simulink model "RadarSimulinkProjectRev003"  (R2024a)
settings: Solver=VariableStepAuto  StartTime=0.0  StopTime=0.012  RelTol=1e-3
values from neighbouring files (symbols this model uses):
  AngleTime = SweepTime/10    (= 10000)    [InitializationOfVariablesRev000.m]    (also in InitializationOfVariablesRev001.m; InitializationOfVariablesRev002.m = 2000; InitializationOfVariablesRev003.m = 20000; InitializationOfVariablesRev004.m = 2097152)
  ASR_LUT = Rsamp    [InitializationOfVariablesRev003.m]    (also in InitializationOfVariablesRev004.m = round((R*2*SystemFs)/c); InitializationOfVariablesRev005.m = round((R*2*SystemFs)/c))
  Btn_Debounce = 20000    [InitializationOfVariablesRev003.m]    (also in InitializationOfVariablesRev004.m; InitializationOfVariablesRev005.m)
  ChirpNc = 128    [InitializationOfVariablesRev004.m]    (also in InitializationOfVariablesRev005.m)
  ChirpSizeLength = length(FCW)    [InitializationOfVariablesRev004.m]    (also in InitializationOfVariablesRev005.m = 16384)
  FreqDeltaPeriod = 54    [InitializationOfVariablesRev003.m]    (also in InitializationOfVariablesRev004.m = 1)
  RXFFTLength = 4096    [InitializationOfVariablesRev003.m]    (also in InitializationOfVariablesRev004.m = 1024; InitializationOfVariablesRev005.m = 2048)
  SweepTime = 100000    [InitializationOfVariablesRev000.m]    (also in InitializationOfVariablesRev001.m; InitializationOfVariablesRev002.m = 20000; InitializationOfVariablesRev003.m = 200000; InitializationOfVariablesRev004.m = 23068672)
undefined symbols (not defined in the file or in its folder): SignalGenerationForAnalysis, Subsystem, xc7a200tfbg676
libraries: hdlBasic x247, hdlDSPIP x12, hdlUtilities x2, vmcUtilities x1
(part 1 of 2)
settings Model: Creator=Cube II  LastModifiedBy=Cube II

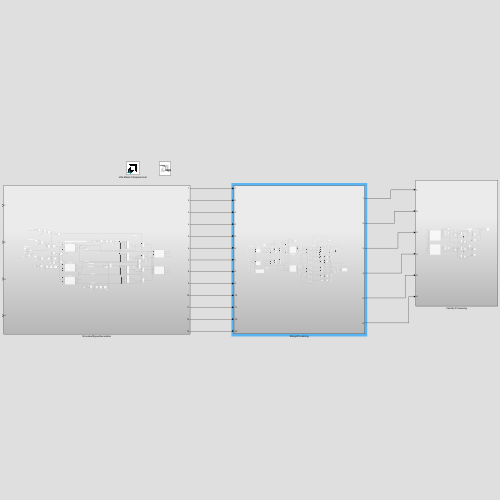
[thumbnail: Simulink's stored preview of the top-level diagram]
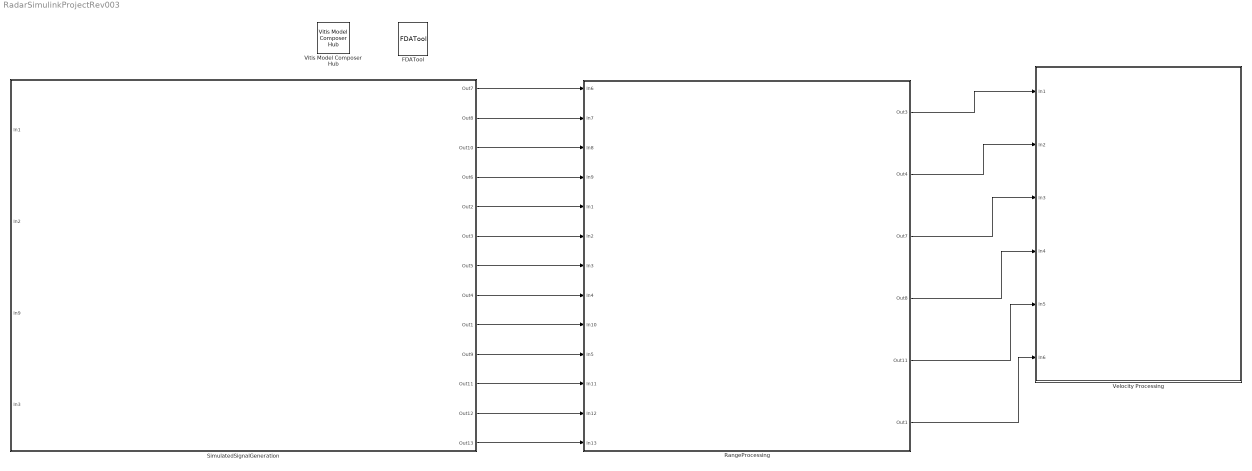
== system RadarSimulinkProjectRev003 ==
  FDATool : hdlUtilities/FDATool  block_type=fdatool
      settings: infoedit=FDATool
  RangeProcessing : Subsystem
  SimulatedSignalGeneration : Subsystem  SystemSampleTime=1/200e6
  Velocity Processing : Subsystem
  Vitis Model Composer Hub : vmcUtilities/Vitis Model Composer Hub  Tag=genX  CodeGeneration=off  SubsystemName=Subsystem  BlockHierPath=SignalGenerationForAnalysis/Subsystem  CompilationType=HDLCompilation  SubsystemType=HDLNode  ExportTypeV2=IP Catalog  StartColumn=1  NumberOfColumns=1  TargetDirectory=./netlist  exportDesign=off  analyzeDesign=on  validateDesignOnHw=off  ExportType=AI Engines  IpVendor=xilinx.com  IpLibrary=hls  IpVersion=1.0  IpHWLanguage=Verilog  AieCompilerOptions={}  AieSimulatorOptions={}  CreateTestbench=on  TestbenchStackSize=10  RunRtlSim=off  RunCSim=off  RunAieSim=off  AieSimTimeout=50000  RunAieSimProfiling=off  LaunchVitisAnalyzer=off  PlotOutput=off  RunX86Sim=off  X86SimTimeout=10  GenHwImage=off  GenLibadfXo=on  GenHwValidationCode=off  PlatformType=Not Specified  HwSystemType=Baremetal  HwValidationTarget=hw  ProjDevice=Artix-7 AC701 Evaluation Platform (xc7a200tfbg676-2)  ProjDevicePart=xc7a200tfbg676-2  AIEType=None  SamplePeriod=-1  ClockFrequency=200  DataPathParallelism=1  xilinxfamily=artix7  part=xc7a200t  speed=-2  package=fbg676  directory=./netlist\ip\Subsystem\src  testbench=off  incr_netlist=off  synthesis_tool=Vivado  clock_wrapper=Clock Enables  dbl_ovrd=According to Block Masks  dcm_input_clock_period=10  sysclk_period=5  simulink_period=1/200e6  eval_field=0  IPInfoJsonString="{\"DUTSubsystemName\":\"Subsystem\",\"HDLSubsystem\":{\"SubsystemName\":\"Subsystem\",\"IPName\":\"Subsystem\",\"IPLibrary\":\"VMC\",\"IPVendor\":\"User Company\",\"IPVersion\":\"1.0\",\"TargetDirectory\":\"./netlist\",\"SubsystemDir\":\"./netlist\\\\ip\\\\Subsystem\",\"FreqHz\":\"200000000\"},\"SubsystemTag\":\"HDLNode\"}"  LogFileName=S:\RadarProjectSimulink\netlist\model_composer.log  NThreads=4  IPConfigFile=C:\Users\Cube II\AppData\Local\Temp\vmctmp-5941030035629153029\SignalGenerationForAnalysis_ipconfig.json
  wires:
  SimulatedSignalGeneration/3(Out10) -> RangeProcessing/3(In8)
  SimulatedSignalGeneration/4(Out6) -> RangeProcessing/4(In9)
  SimulatedSignalGeneration/7(Out5) -> RangeProcessing/7(In3)
  SimulatedSignalGeneration/8(Out4) -> RangeProcessing/8(In4)
  SimulatedSignalGeneration/10(Out9) -> RangeProcessing/10(In5)
  SimulatedSignalGeneration/9(Out1) -> RangeProcessing/9(In10)
  SimulatedSignalGeneration/2(Out8) -> RangeProcessing/2(In7)
  SimulatedSignalGeneration/1(Out7) -> RangeProcessing/1(In6)
  SimulatedSignalGeneration/6(Out3) -> RangeProcessing/6(In2)
  SimulatedSignalGeneration/5(Out2) -> RangeProcessing/5(In1)
  SimulatedSignalGeneration/11(Out11) -> RangeProcessing/11(In11)
  SimulatedSignalGeneration/12(Out12) -> RangeProcessing/12(In12)
  RangeProcessing/1(Out3) -> Velocity Processing/1(In1)
  RangeProcessing/2(Out4) -> Velocity Processing/2(In2)
  RangeProcessing/3(Out7) -> Velocity Processing/3(In3)
  RangeProcessing/4(Out8) -> Velocity Processing/4(In4)
  RangeProcessing/5(Out11) -> Velocity Processing/5(In5)
  RangeProcessing/6(Out1) -> Velocity Processing/6(In6)
  SimulatedSignalGeneration/13(Out13) -> RangeProcessing/13(In13)

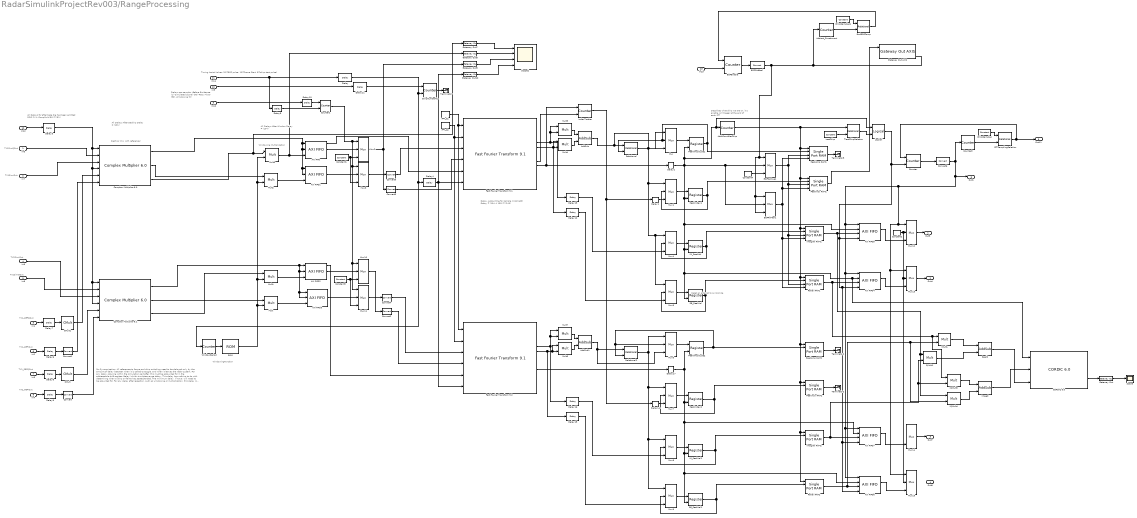
== system RadarSimulinkProjectRev003/RangeProcessing ==
  note: Describes what chirp we are on, it's enable will trigger at the end of each FFT
  note: All Delays for after base Sig has been emitted
      | DDS (1) + CompMult (50) = (51)
  note: Delays per sample:
      | -Before Emittance (1)
      | -Simulated Signal (50)
      | -Recv Mixer (50)
      | -Windowing (3)
  note: TX1SimIOut
  note: TX1SimQOut
  note: TX2SimIOut
  note: TX2SimQOut
  note: TX1_REFIOut
  note: TX1_REFQOut
  note: TX2_REFIOut
  note: TX1_REFQOut
  note: Dechirp (mix with reference)
  note: Timing Assist Values (11=EOF pulse, 10=Frame Start, 9=chirp start pulse)
  note: WindowingFunction
  note: Windowing Multiplication
  note: For Syncronization: All references to frame and chirp switching need to be delayed only by the amount of delay between when it is called to toggle, and when it leaves the radar system.
      |
      | For any delay occuring within the simulation part after, this must be accounted for in the addressable shift register (delay) which simulates range delay. This delay has nothing to do with determinng when a chirp or frame has started/ended. The minimum delay, if not 0, will need to be acounted for.
      |
      | For any delay after reception, such as windowing or multiplication, this delay is relevant to anything that has to do with the processes that depend on knowing when a frame or chirp has started/ended. Since it should only start sampling once a signal theoretically should have arrived from 0 meters (no sim delay)
  note: All Delays After Dechirp
      | Delay = (101)
  note: Delay, accounting for sample missmatch
      | Delay = (104 + 139) = (243)
  note: All Delays After Window
      | Delay = (104)
  note: Reset an attempt to syncronize
  In6 : Inport
  In7 : Inport  Port=2
  In8 : Inport  Port=3
  In9 : Inport  Port=4
  In1 : Inport  Port=5
  In2 : Inport  Port=6
  In3 : Inport  Port=7
  In4 : Inport  Port=8
  In10 : Inport  Port=9
  In5 : Inport  Port=10
  In11 : Inport  Port=11
  In12 : Inport  Port=12
  In13 : Inport  Port=13
  AXI FIFO{,1..3} (4 alike) : hdlBasic/AXI FIFO  input_depth_axis=256  actual_fifo_depth_label=258  enable_tdata=on  enable_tdest=off  enable_tstrb=off  enable_tready=on  enable_tid=off  enable_tuser=off  enable_tkeep=off  enable_tlast=off  has_aresetn=off  enable_data_counts_axis=off  fifo_implementation_type_axis=Common Clock Block RAM  trim_axipin_name=on  programmable_full_type_axis=Full  full_threshold_assert_value_axis=0  programmable_empty_type_axis=Empty  empty_threshold_assert_value_axis=1022  underflow_flag_axi=0  underflow_sense_axi=Active High  overflow_flag_axi=0  overflow_sense_axi=Active High  simulation_type=fast_sim  XmcBlockStatus=1  maskContainerNames=tabcontainer1  block_type=axi_fifo  block_config=sysgen:AXI_FIFO_config
  AXI FIFO{4..7} (4 alike) : hdlBasic/AXI FIFO  input_depth_axis=128  actual_fifo_depth_label=130  enable_tdata=on  enable_tdest=off  enable_tstrb=off  enable_tready=on  enable_tid=off  enable_tuser=off  enable_tkeep=off  enable_tlast=on  has_aresetn=off  enable_data_counts_axis=off  fifo_implementation_type_axis=Common Clock Block RAM  trim_axipin_name=on  programmable_full_type_axis=Full  full_threshold_assert_value_axis=0  programmable_empty_type_axis=Empty  empty_threshold_assert_value_axis=1022  underflow_flag_axi=0  underflow_sense_axi=Active High  overflow_flag_axi=0  overflow_sense_axi=Active High  simulation_type=fast_sim  XmcBlockStatus=1  maskContainerNames=tabcontainer1  block_type=axi_fifo  block_config=sysgen:AXI_FIFO_config
  AddSub : hdlBasic/AddSub  mode=Addition  use_carryin=off  use_carryout=off  en=off  latency=0  precision=Full  arith_type=Unsigned  n_bits=16  bin_pt=14  quantization=Truncate  overflow=Wrap  use_behavioral_HDL=off  hw_selection=Fabric  pipelined=off  XmcBlockStatus=1  maskContainerNames=tabcontainer1  block_type=addsub  block_config=sysgen:Addsub_config
  AddSub1 : hdlBasic/AddSub  mode=Addition  use_carryin=off  use_carryout=off  en=off  latency=0  precision=Full  arith_type=Unsigned  n_bits=16  bin_pt=14  quantization=Truncate  overflow=Wrap  use_behavioral_HDL=off  hw_selection=Fabric  pipelined=off  XmcBlockStatus=1  maskContainerNames=tabcontainer1  block_type=addsub  block_config=sysgen:Addsub_config
  AddrCountPerChirp : hdlBasic/Counter  cnt_type=Count limited  cnt_to=ChirpNc-1  operation=Up  start_count=0  cnt_by_val=1  arith_type=Unsigned  n_bits=7  bin_pt=0  load_pin=off  rst=off  en=on  explicit_period=Explicit  period=1/200e6  use_behavioral_HDL=off  implementation=Fabric  XmcBlockStatus=1  maskContainerNames=group1  block_type=counter  block_config=sysgen:Counter_config  block_width=531  block_height=1023
  Addrcnt_Durationcnt : hdlBasic/Counter  cnt_type=Count limited  cnt_to=ChirpNc-1  operation=Up  start_count=0  cnt_by_val=1  arith_type=Unsigned  n_bits=7  bin_pt=0  load_pin=off  rst=off  en=on  explicit_period=Explicit  period=1/200e6  use_behavioral_HDL=off  implementation=Fabric  XmcBlockStatus=1  maskContainerNames=group1  block_type=counter  block_config=sysgen:Counter_config  block_width=531  block_height=1023
  CMult : hdlBasic/CMult  const=-1  gui_display_data_type=Fixed-point  const_n_bits=1  const_bin_pt=0  float_type=Single  exp_bits=8  fraction_bits=24  en=off  latency=0  precision=Full  arith_type="Signed  (2's comp)"  n_bits=16  bin_pt=14  quantization=Truncate  overflow=Wrap  use_behavioral_HDL=off  mem_type=Distributed RAM  pipeline=off  XmcBlockStatus=1  maskContainerNames=tabcontainer1  block_type=cmult  block_config=sysgen:CMult_config
      settings: infoedit=[]
  CMult1 : hdlBasic/CMult  const=-1  gui_display_data_type=Fixed-point  const_n_bits=1  const_bin_pt=0  float_type=Single  exp_bits=8  fraction_bits=24  en=off  latency=0  precision=Full  arith_type="Signed  (2's comp)"  n_bits=16  bin_pt=14  quantization=Truncate  overflow=Wrap  use_behavioral_HDL=off  mem_type=Distributed RAM  pipeline=off  XmcBlockStatus=1  maskContainerNames=tabcontainer1  block_type=cmult  block_config=sysgen:CMult_config
      settings: infoedit=[]
  CORDIC 6.0 : hdlDSPIP/CORDIC 6.0   functional_selection=Arc_Tan  architectural_configuration=Parallel  pipelining_mode=Maximum  data_format=SignedFraction  phase_format=Radians  input_width=16  output_width=16  round_mode=Truncate  iterations=0  precision=0  compensation_scaling=No_Scale_Compensation  coarse_rotation=on  aclken=off  aresetn=off  out_tready=off  cartesian_has_tuser=off  cartesian_has_tlast=off  cartesian_tuser_width=1  phase_has_tuser=off  phase_has_tlast=off  phase_tuser_width=1  out_tlast_behv=Null  flow_control=NonBlocking  optimize_goal=Resources  trim_axipin_name=on  simulation_type=hybrid_sim  simulation_model=sysgen:cordic_v6_0  data_path_portlist={'s_axis_cartesian_tdata_imag', 's_axis_cartesian_tdata_real', 's_axis_phase_tdata_phase', 'm_axis_dout_tdata_imag', 'm_axis_dout_tdata_real', 'm_axis_dout_tdata_phase','m_axis_dout_tdata'}  ip_name=CORDIC  ip_version=6.0  dsptool_ready=true  ipcore_usecache=true  ipcore_useipmodelcache=true  wrapper_available=true  port_translation_map={ 'aclken' => 'en', 'aresetn' => 'rst' }  XmcBlockStatus=1  maskContainerNames=group15  block_type=cordic_v6_0  block_config=sysgen:rodinimport_config  block_width=800
  ChirpNumberNc : hdlBasic/Counter  cnt_type=Count limited  cnt_to=ChirpNc-1  operation=Up  start_count=0  cnt_by_val=1  arith_type=Unsigned  n_bits=8  bin_pt=0  load_pin=off  rst=on  en=on  explicit_period=Explicit  period=1/200e6  use_behavioral_HDL=off  implementation=Fabric  XmcBlockStatus=1  maskContainerNames=group1  block_type=counter  block_config=sysgen:Counter_config  block_width=531  block_height=1023
  ChirpSamples : hdlBasic/Constant  const=127  gui_display_data_type=Fixed-point  arith_type=Unsigned  n_bits=7  bin_pt=0  preci_type=Single  exp_width=8  frac_width=24  explicit_period=on  period=1/200e6  XmcBlockStatus=1  maskContainerNames=tabcontainer1  block_type=constant  block_config=sysgen:Constant_config
  ChirpSamples1 : hdlBasic/Constant  const=127  gui_display_data_type=Fixed-point  arith_type=Unsigned  n_bits=7  bin_pt=0  preci_type=Single  exp_width=8  frac_width=24  explicit_period=on  period=1/200e6  XmcBlockStatus=1  maskContainerNames=tabcontainer1  block_type=constant  block_config=sysgen:Constant_config
  Complex Multiplier 6.0 : hdlDSPIP/Complex Multiplier 6.0   datatype=integer  hasatlast=off  hasatuser=off  atuserwidth=1  hasbtlast=off  hasbtuser=off  btuserwidth=1  multtype=Use_Mults  optimizegoal=Resources  flowcontrol=NonBlocking  outputwidth=34  roundmode=Truncate  hasctrltlast=off  hasctrltuser=off  ctrltuserwidth=1  outtlastbehv=Null  latencyconfig=Manual  minimumlatency=50  aclken=off  aresetn=off  trim_axipin_name=on  simulation_type=hybrid_sim  simulation_model=sysgen:cmpy_v6_0  data_path_portlist={ 's_axis_a_tdata_real', 's_axis_a_tdata_imag', 's_axis_b_tdata_real', 's_axis_b_tdata_imag', 's_axis_ctrl_tdata_rounding_bit', 'm_axis_dout_tdata_real', 'm_axis_dout_tdata_imag' }  aportwidth=63  bportwidth=63  ip_name=Complex Multiplier  ip_version=6.0  dsptool_ready=true  ipcore_usecache=true  ipcore_useipmodelcache=true  ipcore_verbose=false  ipcore_latency_parameter='minimumlatency'  wrapper_available=true  port_translation_map={ 'aclken' => 'en', 'aresetn' => 'rst'}  XmcBlockStatus=1  maskContainerNames=tabcontainer1  block_type=cmpy_v6_0  block_config=sysgen:rodinimport_config
  Complex Multiplier 6.1 : hdlDSPIP/Complex Multiplier 6.0   datatype=integer  hasatlast=off  hasatuser=off  atuserwidth=1  hasbtlast=off  hasbtuser=off  btuserwidth=1  multtype=Use_Mults  optimizegoal=Resources  flowcontrol=NonBlocking  outputwidth=34  roundmode=Truncate  hasctrltlast=off  hasctrltuser=off  ctrltuserwidth=1  outtlastbehv=Null  latencyconfig=Manual  minimumlatency=50  aclken=off  aresetn=off  trim_axipin_name=on  simulation_type=hybrid_sim  simulation_model=sysgen:cmpy_v6_0  data_path_portlist={ 's_axis_a_tdata_real', 's_axis_a_tdata_imag', 's_axis_b_tdata_real', 's_axis_b_tdata_imag', 's_axis_ctrl_tdata_rounding_bit', 'm_axis_dout_tdata_real', 'm_axis_dout_tdata_imag' }  aportwidth=63  bportwidth=63  ip_name=Complex Multiplier  ip_version=6.0  dsptool_ready=true  ipcore_usecache=true  ipcore_useipmodelcache=true  ipcore_verbose=false  ipcore_latency_parameter='minimumlatency'  wrapper_available=true  port_translation_map={ 'aclken' => 'en', 'aresetn' => 'rst'}  XmcBlockStatus=1  maskContainerNames=tabcontainer1  block_type=cmpy_v6_0  block_config=sysgen:rodinimport_config
  Constant1 : hdlBasic/Constant  const=0  gui_display_data_type=Fixed-point  arith_type=Signed (2's comp)  n_bits=16  bin_pt=15  preci_type=Single  exp_width=8  frac_width=24  explicit_period=on  period=1/200e6  XmcBlockStatus=1  maskContainerNames=tabcontainer1  block_type=constant  block_config=sysgen:Constant_config
  Constant2 : hdlBasic/Constant  const=0  gui_display_data_type=Fixed-point  arith_type=Signed (2's comp)  n_bits=16  bin_pt=15  preci_type=Single  exp_width=8  frac_width=24  explicit_period=on  period=1/200e6  XmcBlockStatus=1  maskContainerNames=tabcontainer1  block_type=constant  block_config=sysgen:Constant_config
  Constant3 : hdlBasic/Constant  const=0  gui_display_data_type=Fixed-point  arith_type=Signed (2's comp)  n_bits=16  bin_pt=15  preci_type=Single  exp_width=8  frac_width=24  explicit_period=on  period=1/200e6  XmcBlockStatus=1  maskContainerNames=tabcontainer1  block_type=constant  block_config=sysgen:Constant_config
  Constant4 : hdlBasic/Constant  const=0  gui_display_data_type=Boolean  arith_type=Boolean  n_bits=16  bin_pt=15  preci_type=Single  exp_width=8  frac_width=24  explicit_period=on  period=1/200e6  XmcBlockStatus=1  maskContainerNames=tabcontainer1  block_type=constant  block_config=sysgen:Constant_config
  Convert : hdlBasic/Convert  gui_display_data_type=Fixed-point  arith_type=Signed (2's comp)  n_bits=17  bin_pt=15  float_type=Single  exp_bits=8  fraction_bits=24  quantization=Truncate  overflow=Wrap  en=off  latency=0  pipeline=off  XmcBlockStatus=1  maskContainerNames=group2  block_type=convert  block_config=sysgen:Convert_config  block_width=595  block_height=885
  Convert1 : hdlBasic/Convert  gui_display_data_type=Fixed-point  arith_type=Signed (2's comp)  n_bits=17  bin_pt=15  float_type=Single  exp_bits=8  fraction_bits=24  quantization=Truncate  overflow=Wrap  en=off  latency=0  pipeline=off  XmcBlockStatus=1  maskContainerNames=group2  block_type=convert  block_config=sysgen:Convert_config  block_width=595  block_height=885
  Convert{2..5} (4 alike) : hdlBasic/Convert  gui_display_data_type=Fixed-point  arith_type=Signed (2's comp)  n_bits=16  bin_pt=15  float_type=Single  exp_bits=8  fraction_bits=24  quantization=Truncate  overflow=Wrap  en=off  latency=0  pipeline=off  XmcBlockStatus=1  maskContainerNames=group2  block_type=convert  block_config=sysgen:Convert_config  block_width=595  block_height=885
  Convert6 : hdlBasic/Convert  gui_display_data_type=Boolean  arith_type=Boolean  n_bits=16  bin_pt=14  float_type=Single  exp_bits=8  fraction_bits=24  quantization=Truncate  overflow=Wrap  en=off  latency=0  pipeline=off  XmcBlockStatus=1  maskContainerNames=group2  block_type=convert  block_config=sysgen:Convert_config  block_width=595  block_height=885
  Counter : hdlBasic/Counter  cnt_type=Count limited  cnt_to=1  operation=Up  start_count=0  cnt_by_val=1  arith_type=Unsigned  n_bits=1  bin_pt=0  load_pin=off  rst=on  en=on  explicit_period=Explicit  period=1/200e6  use_behavioral_HDL=off  implementation=Fabric  XmcBlockStatus=1  maskContainerNames=group1  block_type=counter  block_config=sysgen:Counter_config  block_width=531  block_height=1023
  Counter1 : hdlBasic/Counter  cnt_type=Count limited  cnt_to=1  operation=Up  start_count=0  cnt_by_val=1  arith_type=Unsigned  n_bits=1  bin_pt=0  load_pin=off  rst=on  en=on  explicit_period=Inferred from inputs  period=1  use_behavioral_HDL=off  implementation=Fabric  XmcBlockStatus=1  maskContainerNames=group1  block_type=counter  block_config=sysgen:Counter_config  block_width=531  block_height=1023
  Counter2 : hdlBasic/Counter  cnt_type=Count limited  cnt_to=ChirpNc-1  operation=Up  start_count=0  cnt_by_val=1  arith_type=Unsigned  n_bits=7  bin_pt=0  load_pin=off  rst=off  en=on  explicit_period=Explicit  period=1/200e6  use_behavioral_HDL=off  implementation=Fabric  XmcBlockStatus=1  maskContainerNames=group1  block_type=counter  block_config=sysgen:Counter_config  block_width=531  block_height=1023
  Delay : hdlBasic/Delay  rst=off  en=off  latency=104  reg_retiming=off  XmcBlockStatus=1  maskContainerNames=group1  block_type=delay  block_config=sysgen:Delay_config
  Delay{1,12..16} (6 alike) : hdlBasic/Delay  rst=off  en=off  latency=3  reg_retiming=off  XmcBlockStatus=1  maskContainerNames=group1  block_type=delay  block_config=sysgen:Delay_config
  Delay10 : hdlBasic/Delay  rst=off  en=off  latency=243  reg_retiming=off  XmcBlockStatus=1  maskContainerNames=group1  block_type=delay  block_config=sysgen:Delay_config
  Delay11 : hdlBasic/Delay  rst=off  en=off  latency=104  reg_retiming=off  XmcBlockStatus=1  maskContainerNames=group1  block_type=delay  block_config=sysgen:Delay_config
  Delay17 : hdlBasic/Delay  rst=off  en=off  latency=1  reg_retiming=off  XmcBlockStatus=1  maskContainerNames=group1  block_type=delay  block_config=sysgen:Delay_config
  Delay2 : hdlBasic/Delay  rst=off  en=off  latency=1  reg_retiming=off  XmcBlockStatus=1  maskContainerNames=group1  block_type=delay  block_config=sysgen:Delay_config
  Delay{3,6..9} (5 alike) : hdlBasic/Delay  rst=off  en=off  latency=51  reg_retiming=off  XmcBlockStatus=1  maskContainerNames=group1  block_type=delay  block_config=sysgen:Delay_config
  Delay4 : hdlBasic/Delay  rst=off  en=off  latency=139  reg_retiming=off  XmcBlockStatus=1  maskContainerNames=group1  block_type=delay  block_config=sysgen:Delay_config
  Delay5 : hdlBasic/Delay  rst=off  en=off  latency=104  reg_retiming=off  XmcBlockStatus=1  maskContainerNames=group1  block_type=delay  block_config=sysgen:Delay_config
  EOFCntBool : hdlBasic/Convert  gui_display_data_type=Boolean  arith_type=Boolean  n_bits=16  bin_pt=14  float_type=Single  exp_bits=8  fraction_bits=24  quantization=Truncate  overflow=Wrap  en=off  latency=0  pipeline=off  XmcBlockStatus=1  maskContainerNames=group2  block_type=convert  block_config=sysgen:Convert_config  block_width=595  block_height=885
  EOFEnable : hdlBasic/Counter  cnt_type=Count limited  cnt_to=1  operation=Up  start_count=0  cnt_by_val=1  arith_type=Unsigned  n_bits=1  bin_pt=0  load_pin=off  rst=on  en=on  explicit_period=Explicit  period=1/200e6  use_behavioral_HDL=off  implementation=Fabric  XmcBlockStatus=1  maskContainerNames=group1  block_type=counter  block_config=sysgen:Counter_config  block_width=531  block_height=1023
  EOFRAMen1 : hdlBasic/Mux  inputs=2  en=off  latency=0  precision=Full  arith_type=Unsigned  n_bits=16  bin_pt=14  quantization=Truncate  overflow=Wrap  XmcBlockStatus=1  maskContainerNames=tabcontainer1  block_type=mux  block_config=sysgen:Mux_config
  EOFRAMwe1 : hdlBasic/Mux  inputs=2  en=off  latency=0  precision=Full  arith_type=Unsigned  n_bits=16  bin_pt=14  quantization=Truncate  overflow=Wrap  XmcBlockStatus=1  maskContainerNames=tabcontainer1  block_type=mux  block_config=sysgen:Mux_config
  EndEOFComp : hdlBasic/Relational  mode=a=b  op_type=Bool  en=off  latency=0  XmcBlockStatus=1  maskContainerNames=tabcontainer1  block_type=relational  block_config=sysgen:Relational_config
  FFTSamplingRelation : hdlBasic/Relational  mode=a=b  op_type=Bool  en=off  latency=0  XmcBlockStatus=1  maskContainerNames=tabcontainer1  block_type=relational  block_config=sysgen:Relational_config
  FFT_C1 : hdlBasic/Constant  const=1.0  gui_display_data_type=Fixed-point  arith_type=Unsigned  n_bits=1  bin_pt=0  preci_type=Single  exp_width=8  frac_width=24  explicit_period=on  period=1/200e6  XmcBlockStatus=1  maskContainerNames=tabcontainer1  block_type=constant  block_config=sysgen:Constant_config
  FFT_C2 : hdlBasic/Constant  const=1.0  gui_display_data_type=Boolean  arith_type=Boolean  n_bits=1  bin_pt=0  preci_type=Single  exp_width=8  frac_width=24  explicit_period=on  period=1/200e6  XmcBlockStatus=1  maskContainerNames=tabcontainer1  block_type=constant  block_config=sysgen:Constant_config
  Fast Fourier Transform 9.1 : hdlDSPIP/Fast Fourier Transform 9.1   transform_length=16384  target_clock_frequency=250  target_data_throughput=50  implementation_options=pipelined_streaming_io  run_time_configurable_transform_length=off  enable_ssr=off  super_sample_rates=1  data_format=fixed_point  phase_factor_width=24  scaling_options=block_floating_point  rounding_modes=truncation  aclken=off  aresetn=off  output_ordering=natural_order  cyclic_prefix_insertion=off  throttle_scheme=realtime  xk_index=on  ovflo=off  trim_axipin_name=on  memory_options_data=block_ram  memory_options_phase_factors=block_ram  number_of_stages_using_block_ram_for_data_and_phase_factors=8  memory_options_reorder=block_ram  memory_options_hybrid=off  complex_mult_type=use_mults_resources  butterfly_type=use_xtremedsp_slices  simulation_type=hybrid_sim  simulation_model=sysgen:xfftv9_cmodel  data_path_portlist={ 's_axis_data_tdata', 'm_axis_data_tdata', 'm_axis_status_tdata', 'event_fft_overflow' }  channels=1  input_ordering=natural_order  input_width=16  ip_name=Fast Fourier Transform  ip_version=9.1  dsptool_ready=true  ipcore_usecache=true  ipcore_useipmodelcache=true  wrapper_available=true  port_translation_map={ 'aclken' => 'en', 'aresetn' => 'rst'}  XmcBlockStatus=1  maskContainerNames=tabcontainer1  block_type=xfft_v9_1  block_config=sysgen:rodinimport_config
  Fast Fourier Transform 9.2 : hdlDSPIP/Fast Fourier Transform 9.1   transform_length=16384  target_clock_frequency=250  target_data_throughput=50  implementation_options=pipelined_streaming_io  run_time_configurable_transform_length=off  enable_ssr=off  super_sample_rates=1  data_format=fixed_point  phase_factor_width=24  scaling_options=block_floating_point  rounding_modes=truncation  aclken=off  aresetn=off  output_ordering=natural_order  cyclic_prefix_insertion=off  throttle_scheme=realtime  xk_index=on  ovflo=off  trim_axipin_name=on  memory_options_data=block_ram  memory_options_phase_factors=block_ram  number_of_stages_using_block_ram_for_data_and_phase_factors=8  memory_options_reorder=block_ram  memory_options_hybrid=off  complex_mult_type=use_mults_resources  butterfly_type=use_xtremedsp_slices  simulation_type=hybrid_sim  simulation_model=sysgen:xfftv9_cmodel  data_path_portlist={ 's_axis_data_tdata', 'm_axis_data_tdata', 'm_axis_status_tdata', 'event_fft_overflow' }  channels=1  input_ordering=natural_order  input_width=16  ip_name=Fast Fourier Transform  ip_version=9.1  dsptool_ready=true  ipcore_usecache=true  ipcore_useipmodelcache=true  wrapper_available=true  port_translation_map={ 'aclken' => 'en', 'aresetn' => 'rst'}  XmcBlockStatus=1  maskContainerNames=tabcontainer1  block_type=xfft_v9_1  block_config=sysgen:rodinimport_config
  Gateway Out{,7..10} (5 alike) : hdlBasic/Gateway Out  inherit_from_input=off  bool_to_boolean=off  hdl_port=on  rows=1  columns=1  UseAsDAC=off  DACChannel='1'  interface=None  automatic_assignment=on  address_offset=hex2dec('00')  intf_name=''  intf_description=''  timing_constraint=None  locs_specified=off  LOCs={}  io_standard={}  XmcBlockStatus=1  maskContainerNames=group4  block_type=gatewayout  block_config=sysgen:gateway_out_config  block_width_w=590  block_height_w=620  block_width=620  block_height=750
  Gateway Out AXIS : hdlUtilities/Gateway Out AXIS  mask_sample_period=1  bool_to_boolean=off  block_type=gatewayoutaxi
  IM_PeakVal : hdlBasic/Register  init=0  rst=on  en=off  XmcBlockStatus=1  maskContainerNames=tabcontainer1  block_type=register  block_config=sysgen:Register_config
  IM_PeakVal1 : hdlBasic/Register  init=0  rst=on  en=off  XmcBlockStatus=1  maskContainerNames=tabcontainer1  block_type=register  block_config=sysgen:Register_config
  IMult1 : hdlBasic/Mult  precision=Full  arith_type="Signed  (2's comp)"  n_bits=16  bin_pt=14  quantization=Truncate  overflow=Wrap  en=off  latency=3  opt_float=off  fp_mult_usage=No Usage  use_behavioral_HDL=off  opt=Speed  use_embedded=on  optimum_pipeline=off  pipeline=on  use_rpm=on  placement_style=Triangular  XmcBlockStatus=1  maskContainerNames=group1  block_type=mult  block_config=sysgen:Mult_config  block_width=598  block_height=876
  IQMult3 : hdlBasic/Mult  precision=Full  arith_type="Signed  (2's comp)"  n_bits=16  bin_pt=14  quantization=Truncate  overflow=Wrap  en=off  latency=3  opt_float=off  fp_mult_usage=No Usage  use_behavioral_HDL=off  opt=Speed  use_embedded=on  optimum_pipeline=off  pipeline=on  use_rpm=on  placement_style=Triangular  XmcBlockStatus=1  maskContainerNames=group1  block_type=mult  block_config=sysgen:Mult_config  block_width=598  block_height=876
  IQMult4 : hdlBasic/Mult  precision=Full  arith_type="Signed  (2's comp)"  n_bits=16  bin_pt=14  quantization=Truncate  overflow=Wrap  en=off  latency=3  opt_float=off  fp_mult_usage=No Usage  use_behavioral_HDL=off  opt=Speed  use_embedded=on  optimum_pipeline=off  pipeline=on  use_rpm=on  placement_style=Triangular  XmcBlockStatus=1  maskContainerNames=group1  block_type=mult  block_config=sysgen:Mult_config  block_width=598  block_height=876
  ImagC : hdlBasic/AddSub  mode=Subtraction  use_carryin=off  use_carryout=off  en=off  latency=1  precision=Full  arith_type=Unsigned  n_bits=16  bin_pt=14  quantization=Truncate  overflow=Wrap  use_behavioral_HDL=off  hw_selection=Fabric  pipelined=off  XmcBlockStatus=1  maskContainerNames=tabcontainer1  block_type=addsub  block_config=sysgen:Addsub_config
  ImagVal RAM1 : hdlBasic/Single Port RAM  depth=ChirpNc  initVector=0  distributed_mem=Block RAM  write_mode=Read After Write  rst=off  init_reg=0  en=on  optimize_latency=off  latency=1  optimize=Area  dbl_ovrd=off  simulation_type=fast_sim  XmcBlockStatus=1  maskContainerNames=tabcontainer1  block_type=spram  block_config=sysgen:SPRAM_config
  ImagVal RAM2 : hdlBasic/Single Port RAM  depth=ChirpNc  initVector=0  distributed_mem=Block RAM  write_mode=Read After Write  rst=off  init_reg=0  en=on  optimize_latency=off  latency=1  optimize=Area  dbl_ovrd=off  simulation_type=fast_sim  XmcBlockStatus=1  maskContainerNames=tabcontainer1  block_type=spram  block_config=sysgen:SPRAM_config
  IndexTracker : hdlBasic/Counter  cnt_type=Count limited  cnt_to=RXFFTLength-1  operation=Up  start_count=0  cnt_by_val=1  arith_type=Unsigned  n_bits=14  bin_pt=0  load_pin=off  rst=on  en=on  explicit_period=Explicit  period=1/200e6  use_behavioral_HDL=off  implementation=Fabric  XmcBlockStatus=1  maskContainerNames=group1  block_type=counter  block_config=sysgen:Counter_config  block_width=531  block_height=1023
  LastChirp : hdlBasic/Constant  const=0  gui_display_data_type=Fixed-point  arith_type=Unsigned  n_bits=7  bin_pt=0  preci_type=Single  exp_width=8  frac_width=24  explicit_period=on  period=1/200e6  XmcBlockStatus=1  maskContainerNames=tabcontainer1  block_type=constant  block_config=sysgen:Constant_config
  Logical : hdlBasic/Logical  logical_function=AND  inputs=2  en=off  latency=0  precision=Full  arith_type=Unsigned  n_bits=16  bin_pt=0  align_bp=on  overflow=[]  quantization=[]  XmcBlockStatus=1  maskContainerNames=tabcontainer1  block_type=logical  block_config=sysgen:Logical_config
  Mult{,1..7} (8 alike) : hdlBasic/Mult  precision=Full  arith_type="Signed  (2's comp)"  n_bits=16  bin_pt=14  quantization=Truncate  overflow=Wrap  en=off  latency=3  opt_float=off  fp_mult_usage=No Usage  use_behavioral_HDL=off  opt=Speed  use_embedded=on  optimum_pipeline=off  pipeline=on  use_rpm=on  placement_style=Triangular  XmcBlockStatus=1  maskContainerNames=group1  block_type=mult  block_config=sysgen:Mult_config  block_width=598  block_height=876
  Mux{,1..15} (16 alike) : hdlBasic/Mux  inputs=2  en=off  latency=0  precision=Full  arith_type=Unsigned  n_bits=16  bin_pt=14  quantization=Truncate  overflow=Wrap  XmcBlockStatus=1  maskContainerNames=tabcontainer1  block_type=mux  block_config=sysgen:Mux_config
  PeakAmp RAM1 : hdlBasic/Single Port RAM  depth=ChirpNc  initVector=0  distributed_mem=Block RAM  write_mode=Read After Write  rst=off  init_reg=0  en=on  optimize_latency=off  latency=1  optimize=Area  dbl_ovrd=off  simulation_type=fast_sim  XmcBlockStatus=1  maskContainerNames=tabcontainer1  block_type=spram  block_config=sysgen:SPRAM_config
  PeakAmp RAM2 : hdlBasic/Single Port RAM  depth=ChirpNc  initVector=0  distributed_mem=Block RAM  write_mode=Read After Write  rst=off  init_reg=0  en=on  optimize_latency=off  latency=1  optimize=Area  dbl_ovrd=off  simulation_type=fast_sim  XmcBlockStatus=1  maskContainerNames=tabcontainer1  block_type=spram  block_config=sysgen:SPRAM_config
  PeakAmplitude1 : hdlBasic/Register  init=0  rst=on  en=off  XmcBlockStatus=1  maskContainerNames=tabcontainer1  block_type=register  block_config=sysgen:Register_config
  PeakAmplitude2 : hdlBasic/Register  init=0  rst=on  en=off  XmcBlockStatus=1  maskContainerNames=tabcontainer1  block_type=register  block_config=sysgen:Register_config
  PeakIndex1 : hdlBasic/Register  init=0  rst=on  en=off  XmcBlockStatus=1  maskContainerNames=tabcontainer1  block_type=register  block_config=sysgen:Register_config
  PeakIndex2 : hdlBasic/Register  init=0  rst=on  en=off  XmcBlockStatus=1  maskContainerNames=tabcontainer1  block_type=register  block_config=sysgen:Register_config
  PeakIndx RAM1 : hdlBasic/Single Port RAM  depth=ChirpNc  initVector=0  distributed_mem=Block RAM  write_mode=Read After Write  rst=off  init_reg=0  en=on  optimize_latency=off  latency=1  optimize=Area  dbl_ovrd=off  simulation_type=fast_sim  XmcBlockStatus=1  maskContainerNames=tabcontainer1  block_type=spram  block_config=sysgen:SPRAM_config
  PeakIndx RAM2 : hdlBasic/Single Port RAM  depth=ChirpNc  initVector=0  distributed_mem=Block RAM  write_mode=Read After Write  rst=off  init_reg=0  en=on  optimize_latency=off  latency=1  optimize=Area  dbl_ovrd=off  simulation_type=fast_sim  XmcBlockStatus=1  maskContainerNames=tabcontainer1  block_type=spram  block_config=sysgen:SPRAM_config
  QMult1 : hdlBasic/Mult  precision=Full  arith_type="Signed  (2's comp)"  n_bits=16  bin_pt=14  quantization=Truncate  overflow=Wrap  en=off  latency=3  opt_float=off  fp_mult_usage=No Usage  use_behavioral_HDL=off  opt=Speed  use_embedded=on  optimum_pipeline=off  pipeline=on  use_rpm=on  placement_style=Triangular  XmcBlockStatus=1  maskContainerNames=group1  block_type=mult  block_config=sysgen:Mult_config  block_width=598  block_height=876
  RE_PeakVal : hdlBasic/Register  init=0  rst=on  en=off  XmcBlockStatus=1  maskContainerNames=tabcontainer1  block_type=register  block_config=sysgen:Register_config
  RE_PeakVal1 : hdlBasic/Register  init=0  rst=on  en=off  XmcBlockStatus=1  maskContainerNames=tabcontainer1  block_type=register  block_config=sysgen:Register_config
  ROM : hdlBasic/ROM  depth=ChirpSizeLength  initVector=WindowCoefficients  distributed_mem=Block RAM  rst=off  init_reg=0  en=off  latency=1  gui_display_data_type=Fixed-point  arith_type=Unsigned  n_bits=16  bin_pt=16  preci_type=Single  exp_width=8  frac_width=24  optimize=Area  use_rpm=on  simulation_type=fast_sim  XmcBlockStatus=1  maskContainerNames=tabcontainer1  block_type=sprom  block_config=sysgen:SPROM_config
  ReVal RAM1 : hdlBasic/Single Port RAM  depth=ChirpNc  initVector=0  distributed_mem=Block RAM  write_mode=Read After Write  rst=off  init_reg=0  en=on  optimize_latency=off  latency=1  optimize=Area  dbl_ovrd=off  simulation_type=fast_sim  XmcBlockStatus=1  maskContainerNames=tabcontainer1  block_type=spram  block_config=sysgen:SPRAM_config
  ReVal RAM2 : hdlBasic/Single Port RAM  depth=ChirpNc  initVector=0  distributed_mem=Block RAM  write_mode=Read After Write  rst=off  init_reg=0  en=on  optimize_latency=off  latency=1  optimize=Area  dbl_ovrd=off  simulation_type=fast_sim  XmcBlockStatus=1  maskContainerNames=tabcontainer1  block_type=spram  block_config=sysgen:SPRAM_config
  RealC : hdlBasic/AddSub  mode=Addition  use_carryin=off  use_carryout=off  en=off  latency=1  precision=Full  arith_type=Unsigned  n_bits=16  bin_pt=14  quantization=Truncate  overflow=Wrap  use_behavioral_HDL=off  hw_selection=Fabric  pipelined=off  XmcBlockStatus=1  maskContainerNames=tabcontainer1  block_type=addsub  block_config=sysgen:Addsub_config
  Relational : hdlBasic/Relational  mode=a>b  op_type=Bool  en=off  latency=0  XmcBlockStatus=1  maskContainerNames=tabcontainer1  block_type=relational  block_config=sysgen:Relational_config
  Relational2 : hdlBasic/Relational  mode=a>b  op_type=Bool  en=off  latency=0  XmcBlockStatus=1  maskContainerNames=tabcontainer1  block_type=relational  block_config=sysgen:Relational_config
  Scope : Scope
  Scope2 : Scope  NumInputPorts=4
  Terminator{,1..3} (4 alike) : Terminator
  TlastChirpRelation : hdlBasic/Relational  mode=a=b  op_type=Bool  en=off  latency=0  XmcBlockStatus=1  maskContainerNames=tabcontainer1  block_type=relational  block_config=sysgen:Relational_config
  WindowPeriod : hdlBasic/Counter  cnt_type=Count limited  cnt_to=ChirpSizeLength-1  operation=Up  start_count=0  cnt_by_val=1  arith_type=Unsigned  n_bits=14  bin_pt=0  load_pin=off  rst=on  en=off  explicit_period=Explicit  period=1/200e6  use_behavioral_HDL=off  implementation=Fabric  XmcBlockStatus=1  maskContainerNames=group1  block_type=counter  block_config=sysgen:Counter_config  block_width=531  block_height=1023
  Out3 : Outport
  Out4 : Outport  Port=2
  Out7 : Outport  Port=3
  Out8 : Outport  Port=4
  Out11 : Outport  Port=5
  Out1 : Outport  Port=6
  wires:
  WindowPeriod/1 -> ROM/1
  In4/1 -> Delay9/1
  In3/1 -> Delay8/1
  In2/1 -> Delay6/1
  In1/1 -> Delay7/1
  In10/1 -> Delay10/1
  FFT_C1/1 -> Fast Fourier Transform 9.2/1, Fast Fourier Transform 9.1/1
  CMult1/1 -> Complex Multiplier 6.0/5
  Convert1/1 -> Complex Multiplier 6.0/6
  In9/1 -> Complex Multiplier 6.1/3
  In8/1 -> Complex Multiplier 6.1/2
  CMult/1 -> Complex Multiplier 6.1/5
  Convert/1 -> Complex Multiplier 6.1/6
  Complex Multiplier 6.1/2 -> Mult/1  "TX2Q"
  Complex Multiplier 6.1/3 -> Mult1/1  "TX2I"
  Delay7/1 -> CMult1/1
  Delay6/1 -> Convert1/1
  Delay8/1 -> CMult/1
  Delay9/1 -> Convert/1
  In12/1 -> Delay3/1
  In6/1 -> Complex Multiplier 6.0/2
  In7/1 -> Complex Multiplier 6.0/3
  In5/1 -> Delay11/1
  FFT_C2/1 -> Fast Fourier Transform 9.1/2, Fast Fourier Transform 9.2/2
  In11/1 -> Delay5/1, Delay/1
  Fast Fourier Transform 9.1/6 -> Mult4/1, Mult4/2, Delay12/1
  PeakAmplitude1/1 -> Relational/2, Mux/2, PeakAmp RAM1/2
  Mux/1 -> PeakAmplitude1/1
  Mux1/1 -> PeakIndex1/1
  Fast Fourier Transform 9.1/10 -> Delay2/1, IndexTracker/1
  Fast Fourier Transform 9.1/9 -> IndexTracker/2
  Delay1/1 -> Mux1/3
  PeakIndex1/1 -> PeakIndx RAM1/2, Mux1/2
  Gateway Out10/1 -> Scope2/4
  Gateway Out9/1 -> Scope2/3
  Gateway Out7/1 -> Scope2/1
  Gateway Out8/1 -> Scope2/2
  Convert5/1 -> Fast Fourier Transform 9.1/3
  Convert3/1 -> Fast Fourier Transform 9.1/4
  Complex Multiplier 6.0/2 -> Mult2/1
  Mult3/1 -> Gateway Out8/1, AXI FIFO/3
  Delay3/1 -> Complex Multiplier 6.1/4, Complex Multiplier 6.1/1, Complex Multiplier 6.0/4, Complex Multiplier 6.0/1
  ROM/1 -> Mult3/2, Mult2/2, Mult1/2, Mult/2
  Delay/1 -> WindowPeriod/1, Delay4/1, ChirpNumberNc/2
  AddSub/1 -> Relational/1, Mux/3
  Fast Fourier Transform 9.1/5 -> Delay13/1, Mult5/2, Mult5/1
  Mult5/1 -> AddSub/1
  Mult4/1 -> AddSub/2
  Complex Multiplier 6.0/1 -> AXI FIFO1/2, AXI FIFO1/1, AXI FIFO/2, AXI FIFO/1
  AXI FIFO/1 -> Fast Fourier Transform 9.1/5
  Delay10/1 -> Counter1/1
  AXI FIFO/2 -> Mux2/2
  Mux2/1 -> Convert3/1, Gateway Out9/1
  Mult2/1 -> AXI FIFO1/3
  Constant1/1 -> Mux3/3, Mux2/3
  AXI FIFO1/2 -> Mux3/2
  Mux3/1 -> Convert5/1
  Complex Multiplier 6.0/3 -> Gateway Out7/1, Mult3/1
  Delay4/1 -> Fast Fourier Transform 9.2/6, Gateway Out10/1, Fast Fourier Transform 9.1/6
  Delay5/1 -> Counter1/2
  Delay11/1 -> ChirpNumberNc/1
  Mux4/1 -> IM_PeakVal/1
  IM_PeakVal/1 -> ImagVal RAM1/2, Mux4/2
  Delay13/1 -> Mux4/3
  Relational/1 -> Mux5/1, Mux4/1, Mux1/1, Mux/1
  RE_PeakVal/1 -> ReVal RAM1/2, Mux5/2
  Mux5/1 -> RE_PeakVal/1
  Delay12/1 -> Mux5/3
  Delay15/1 -> Mux9/3
  Mux9/1 -> RE_PeakVal1/1
  RE_PeakVal1/1 -> ReVal RAM2/2, Mux9/2
  IM_PeakVal1/1 -> ImagVal RAM2/2, Mux8/2
  Relational2/1 -> Mux9/1, Mux8/1, Mux7/1, Mux6/1
  IndexTracker/1 -> Delay14/1, Delay1/1
  Mux8/1 -> IM_PeakVal1/1
  Fast Fourier Transform 9.2/5 -> Delay16/1, Mult7/1, Mult7/2
  Mult6/1 -> AddSub1/2
  Mult7/1 -> AddSub1/1
  AddrCountPerChirp/1 -> ReVal RAM2/1, ImagVal RAM2/1, PeakIndx RAM2/1, PeakAmp RAM2/1, ReVal RAM1/1, ImagVal RAM1/1, PeakIndx RAM1/1, PeakAmp RAM1/1, TlastChirpRelation/1
  Delay17/1 -> PeakAmplitude2/2, AXI FIFO7/2, AXI FIFO6/2, RE_PeakVal1/2, IM_PeakVal1/2, PeakIndex2/2
  Fast Fourier Transform 9.2/6 -> Delay15/1, Mult6/1, Mult6/2
  Fast Fourier Transform 9.2/10 -> Delay17/1
  Mux7/1 -> PeakIndex2/1
  AddSub1/1 -> Mux6/3, Relational2/1
  Mux6/1 -> PeakAmplitude2/1
  PeakAmplitude2/1 -> PeakAmp RAM2/2, Relational2/2, Mux6/2
  Delay14/1 -> Mux7/3
  Delay16/1 -> Mux8/3
  PeakIndex2/1 -> PeakIndx RAM2/2, Mux7/2
  Mux10/1 -> Convert2/1
  Mux11/1 -> Convert4/1
  Counter1/1 -> Mux3/1, Mux11/1, Mux10/1, Mux2/1
  AXI FIFO2/2 -> Mux10/2
  Constant3/1 -> Mux11/3, Mux10/3
  AXI FIFO2/1 -> Fast Fourier Transform 9.2/5
  AXI FIFO3/2 -> Mux11/2
  Mult/1 -> AXI FIFO3/3
  Mult1/1 -> AXI FIFO2/3
  Complex Multiplier 6.1/1 -> AXI FIFO3/1, AXI FIFO3/2, AXI FIFO2/2, AXI FIFO2/1
  Convert4/1 -> Fast Fourier Transform 9.2/3
  Convert2/1 -> Fast Fourier Transform 9.2/4
  ImagVal RAM1/1 -> AXI FIFO5/3, IQMult4/1, QMult1/1  "ImagVal1"
  ReVal RAM1/1 -> IQMult3/1, IMult1/1, AXI FIFO4/3  "ReVal1"
  PeakAmp RAM2/1 -> Terminator1/1  "MAGPeak2"
  ImagVal RAM2/1 -> AXI FIFO7/3, IQMult3/2, QMult1/2  "ImagVal2"
  PeakIndx RAM2/1 -> Terminator2/1  "Peakindx2"
  ReVal RAM2/1 -> AXI FIFO6/3, IQMult4/2, IMult1/2  "ReVal2"
  LastChirp/1 -> TlastChirpRelation/2
  AXI FIFO4/2 -> Mux13/3
  AXI FIFO5/2 -> Mux12/3
  Logical/1 -> Counter/2, AXI FIFO6/4, AXI FIFO7/4, AXI FIFO4/4, AXI FIFO5/4  "TLast"
  TlastChirpRelation/1 -> Logical/2  "TLast"
  Delay2/1 -> EOFRAMen1/2, EOFRAMwe1/2, PeakAmplitude1/2, Logical/1, AddrCountPerChirp/1, AXI FIFO5/2, IM_PeakVal/2, CORDIC 6.0/1, AXI FIFO4/2, RE_PeakVal/2, PeakIndex1/2
  Counter/1 -> Convert6/1
  Counter2/1 -> FFTSamplingRelation/2
  ChirpSamples/1 -> FFTSamplingRelation/1
  FFTSamplingRelation/1 -> Out11/1, Counter/1  "TLast"
  Mux12/1 -> Out3/1
  Mux13/1 -> Out4/1
  ChirpNumberNc/1 -> Terminator/1  "Chirp Number"
  PeakAmp RAM1/1 -> Terminator3/1  "MAGPeak1"
  Constant2/1 -> Mux15/2, Mux13/2, Mux12/2
  Convert6/1 -> Out1/1, Mux15/1, Mux13/1, Mux12/1, AXI FIFO6/1, AXI FIFO7/1, AXI FIFO4/1, AXI FIFO5/1, Counter2/1
  AXI FIFO7/2 -> Mux14/3
  AXI FIFO6/2 -> Mux15/3
  Mux14/1 -> Out7/1
  IMult1/1 -> RealC/1
  QMult1/1 -> RealC/2
  IQMult3/1 -> ImagC/1
  IQMult4/1 -> ImagC/2
  RealC/1 -> CORDIC 6.0/3
  ImagC/1 -> CORDIC 6.0/2
  CORDIC 6.0/2 -> Gateway Out/1
  Gateway Out/1 -> Scope/1
  EOFRAMwe1/1 -> PeakAmp RAM1/3, ReVal RAM1/3, ImagVal RAM1/3, PeakIndx RAM1/3
  EOFRAMen1/1 -> ReVal RAM1/4, ImagVal RAM1/4, PeakIndx RAM1/4, PeakAmp RAM1/4
  EOFCntBool/1 -> Gateway Out AXIS/3, Addrcnt_Durationcnt/1, EOFRAMen1/3, EOFRAMen1/1, EOFRAMwe1/1
  In13/1 -> EOFEnable/2
  PeakIndx RAM1/1 -> Gateway Out AXIS/1  "PeakIndx1"
  Addrcnt_Durationcnt/1 -> EndEOFComp/2
  EOFEnable/1 -> EOFCntBool/1
  ChirpSamples1/1 -> EndEOFComp/1
  EndEOFComp/1 -> EOFEnable/1  "TLast"
  Constant4/1 -> EOFRAMwe1/3
